simulink model "btTest"  (R2015b)
settings: Solver=FixedStepDiscrete  StartTime=0.0  StopTime=Inf  RelTol=1e-3
libraries: freescalecupcompanionlib x1, bluetoothLibrary x1
settings Model: SimulationMode=external  ExtModeTrigDuration=5  Creator=dc315  LastModifiedBy=dc315
settings OptimizationCC: OptimizeModelRefInitCode=on  LifeSpan=1  MaxStackSize=64
settings HardwareCC: ProdBitPerPointer=32  ProdLargestAtomicInteger=Long  ProdLargestAtomicFloat=Double  ProdWordSize=32  ProdHWDeviceType=ARM Compatible->ARM Cortex
settings RTWCC: SystemTargetFile=ert.tlc  TemplateMakefile=ert_default_tmf  Description=Embedded Coder  Toolchain=GNU Tools for ARM Embedded Processors
settings CodeAppCC: IgnoreCustomStorageClasses=off

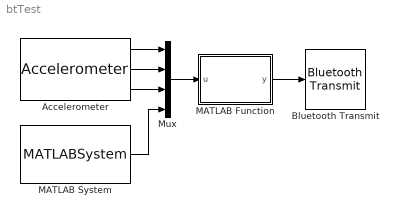
== system btTest ==
  Accelerometer : freescalecupcompanionlib/Accelerometer  SampleTime=0.01
  Bluetooth Transmit : bluetoothLibrary/Bluetooth Transmit  baudRate=9600
  MATLAB Function : MATLAB Function  TreatAsAtomicUnit=on
  MATLAB System : MATLABSystem  System=freedomboard.rpmSensor  SimulateUsing=Code generation
      mask Type: freedomboard.rpmSensor
      mask Display:
      | disp('rpmSensor');
      | port_label('output',1,'rpm');
  Mux : Mux
  wires:
  Mux/1 -> MATLAB Function/1(u)
  Accelerometer/1 -> Mux/1
  Accelerometer/2 -> Mux/2
  Accelerometer/3 -> Mux/3
  MATLAB Function/1(y) -> Bluetooth Transmit/1
  MATLAB System/1 -> Mux/4

== matlab function btTest/MATLAB Function ==
  data: u input; y output
function y = fcn(u)
%#codegen

y = typecast(u,'uint8');
